simulink model "AUAV_V3_TestSensors"  (R2015a)
settings: Solver=FixedStepDiscrete  StartTime=0.0  StopTime=10.0  FixedStep=T  RelTol=1e-3
PreLoadFcn:
  | %T = 0.0025;
  | MavlinkBus;
  | mcuInit;
  | % Baro Altitude Computation
  | % =========================
  | basePressure = 98192.64;
  | baseTemp = 288.215;
  | lapseRate = -0.00198122;
  | baseHeight = 0;
undefined symbols (not defined in the file): A0, A14, A15, A2, A3, A4, A5, A6, accBiasRateLimit, apSampleTime, B0, bankCommandLimit, barAdjust, baroCutoff, baroCutTemp, baroOffset, baroScale, barTGain1, barTGain2, barTMean1, barTMean2, bda, bde, bdr, bdt, bICda, bICde, bICdr, bICdt, cubeAccelGain16405, cubeGyroGain16405, cubeMagGain16405, D0, D11, D7, D8, daLimit, data, daTrimMax, daTrimMin, deLimit, derivativesConstant, deTrimMax, deTrimMin, drLimit, drTrimMax, drTrimMin, dtLimit, dtTrimMax, dtTrimMin, F2, F3, G0, G13, G15, gaind, GS_location, gyroBiasRateLimit, IC1max, imuOffset_xacc ... (+77)
libraries: MCHP_Blockset x158, simulink x84, SLUGS_Library x31, aerolibconvert2 x6, aerolibutil x4, aerolibtransform2 x3, dspmtrx3 x2, aerolibobsolete x2
(part 11 of 23)

== system AUAV_V3_TestSensors/Trim Vals [updated 4.28.16]/Mean Filter the Transition ==
  Failsafe : Inport
  Buffer Failsafe Channel : MATLAB Function  TreatAsAtomicUnit=on
  Choose the Median [navSupport.c] [updated 5.1.16] : MCHP_Blockset/User Functions/C Function Call  ParseFilesChkbx=off  ListFunctions1=Custom Function  Function1=extern uint16_T meanFilter5(uint16_T *u1);  AddHeaderDeclaration=on  Function1Type=when block is updated (default)  Fct1BlockIn=u1  FctReturnBlockOut=on  DataCollected=0  ORDERING=None  SampleTime=-1  MCHP_MASTERLINK=|  PinDigitalInput=[]  PinDigitalOutput=[]  PinAnalogInput=[]
      | AUAV_V3_TestSensors/Microchip Master
      | AUAV V3 Board
      | Busy Flag on D2 (RA6)
  filtered : Outport
  wires:
  Choose the Median [navSupport.c] [updated 5.1.16]/1 -> filtered/1
  Failsafe/1 -> Buffer Failsafe Channel/1(latest)
  Buffer Failsafe Channel/1(history) -> Choose the Median [navSupport.c] [updated 5.1.16]/1

== system AUAV_V3_TestSensors/Update PWM Commands and Send Telemetry [updated 4.27.16]/Convert to Microseconds ==
  PWM : Inport
  Convert to Microseconds : Gain  Gain=0.2
  Data Type Conversion : DataTypeConversion  OutDataTypeStr=uint16
  uS : Outport
  wires:
  Data Type Conversion/1 -> uS/1
  PWM/1 -> Convert to Microseconds/1
  Convert to Microseconds/1 -> Data Type Conversion/1

== system AUAV_V3_TestSensors/Update PWM Commands and Send Telemetry [updated 4.27.16]/Generate PWM Signals Based on the Control Type ==
  note: Navigation Modes:
      | 2 -> PT
      | 3 -> Waypoint
      | 4 -> Mid Level
      | 8-> Sel PT
      | 9-> ISR
      | 10 -> Line Patrol
  PWM(rad) : Inport
  Pilot Console (IC) : Inport  Port=2
  isManual? : Inport  Port=3
  Nav Mode : Inport  Port=4
  Data Type Conversion : DataTypeConversion  OutDataTypeStr=uint16
  Data Type Conversion1 : DataTypeConversion  OutDataTypeStr=uint8
  If : If  NumInputs=2  IfExpression=u2 == 1  ElseIfExpressions=((u1 == 3) | (u1 == 4) | (u1 == 9) | (u1 == 10)), u1 == 2, u1 == 8  ShowElse=off  SampleTime=.01
  If  Control Type Is Manual : Subsystem  TreatAsAtomicUnit=on
  If  Control Type Is Passthrough : Subsystem  TreatAsAtomicUnit=on
  If  Control Type Is Selective Passthrough : Subsystem  TreatAsAtomicUnit=on
  "If  Control Type Is Wp, ISR, LP or  Mid Lvl Cmds" : Subsystem  TreatAsAtomicUnit=on
  Merge : Merge  Inputs=4
  PWM : Outport
  wires:
  If/1 -> If  Control Type Is Manual/Action
  If/2 -> "If  Control Type Is Wp, ISR, LP or  Mid Lvl Cmds"/Action
  If/3 -> If  Control Type Is Passthrough/Action
  If/4 -> If  Control Type Is Selective Passthrough/Action
  If  Control Type Is Manual/1(PWM) -> Merge/1
  "If  Control Type Is Wp, ISR, LP or  Mid Lvl Cmds"/1(PWM (abs)) -> Merge/2
  If  Control Type Is Passthrough/1(PWM (abs)) -> Merge/3
  If  Control Type Is Selective Passthrough/1(PWM) -> Merge/4
  PWM(rad)/1 -> "If  Control Type Is Wp, ISR, LP or  Mid Lvl Cmds"/1(PWM(rad)), If  Control Type Is Selective Passthrough/1(PWM(rad))
  Pilot Console (IC)/1 -> If  Control Type Is Manual/1(Pilot (IC)), If  Control Type Is Passthrough/1(Pilot (IC)), If  Control Type Is Selective Passthrough/2(Pilot (IC))
  Data Type Conversion/1 -> PWM/1
  isManual?/1 -> If/2
  Nav Mode/1 -> Data Type Conversion1/1
  Data Type Conversion1/1 -> If/1
  Merge/1 -> Data Type Conversion/1

== system AUAV_V3_TestSensors/Update PWM Commands and Send Telemetry [updated 4.27.16]/Send_Cmd_6DOF_HIL ==
  Enable : EnablePort
  COMP_ID : Constant  OutDataTypeStr=uint8
  Get Raw Commands : DataStoreRead  DialogController=Simulink.DDGSource  DataStoreName=mlPwmCommands  DataStoreElements=mlPwmCommands
  Get time5 : DataStoreRead  DataStoreName=time_since_boot_usec  DataStoreElements=time_since_boot_usec
  PackRawServo : MCHP_Blockset/User Functions/C Function Call  ParseFilesChkbx=on  ListFunctions1=Custom Function  Function1=uint16_t HIL_PackRawServo(uint8_t system_id, uint8_t component_id, mavlink_servo_output_raw_t mlPwmCommands ,uint32_t time_usec)  AddHeaderDeclaration=on  Function1Type=when block is updated (default)  Fct1BlockIn="system_id  , component_id  , mlPwmCommands  , time_usec"  FctReturnBlockOut=on  DataCollected="s.chksm=reshape({ '638503-Feb-2015 20:58:10','251913-Sep-2016 12:15:14','1628414-Sep-2016 10:06:29','3754120-Sep-2016 10:12:03','360317-Jun-2016 15:34:16','7114620-Sep-2016 10:38:54','954931-Aug-2016 15:03:40','295520-Sep-2016 10:30:42','268124-Jun-2016 00:23:34','556017-Jun-2016 15:34:16','963217-Jun-2016 15:34:16','1086024-Jun-2016 00:23:34','372414-Sep-2016 14:01:55','998814-Sep-2016 11:55:45','509015-Sep-2016 09:12:19'},1,15);s.File1=reshape({ '  void  newCircBuffer(CBRef cB)','  void  freeCircBuffer(CBRef* cB)','  void  freeCircBuffer(CBRef* cB)',' unsigned int  getLength(CBRef cB)','  int  readHead(CBRef cB)','  int  readTail(CBRef cB)',' unsigned char  peak(CBRef cB)',' unsigned char  readFront(CBRef cB)',' unsigned char  writeBack(CBRef cB, unsigned char data)','  void  makeEmpty(CBRef cB)','  void  printCircBuf(CBRef cB)'},1,11);s.File2=reshape({ '  void  uartBufferInit(void)','  void  __attribute__((__interrupt__, no_auto_psv)) _U4RXInterrupt(void)','  void  getGPSRawData(unsigned char* gpsBuffer)',' unsigned char  isGPSNovatel(void)'},1,4);s.File3=reshape({ '  char  hex2char(char halfhex)','  float  degMinToDeg(unsigned char degrees, float minutes)',' unsigned char  gpsUbloxSeparate(unsigned char* outStream)','  void  gpsUbloxParse(void)','  void  getGpsUbloxMainData(float* data)','  char  gpSmbl(char symbl)',' unsigned char  myTokenizer(char* stringToTokenize, char token, char * returnToken)','  void  parseRMC(unsigned char* stream)','  void  parseGGA(unsigned char* stream)',' unsigned char  getChecksum(unsigned char* sentence, unsigned char size)','  void  gpsDebugMsg(unsigned char buf)'},1,11);s.File4=reshape({ '  void  uartMavlinkBufferInit(void)','  void __attribute__((__interrupt__,__auto_psv__)) _U1RXInterrupt(void)','  uint8_t  isFinite(float s)','  void  InitParameterInterface(void)','  void  protDecodeMavlink(void)','  uint16_t  MissionInterfaceResponse(uint8_t system_id, uint8_t component_id)','  uint16_t  ParameterInterfaceResponse(uint8_t system_id, uint8_t component_id)','  uint16_t  PackHeartBeat(uint8_t system_id, uint8_t component_id)','  uint16_t  PackTextMsg(uint8_t system_id, uint8_t component_id, unsigned char buf)','  uint16_t  PackRawIMU(uint8_t system_id, uint8_t component_id, mavlink_raw_imu_t mlRawIMUData ,uint32_t time_usec)','  uint16_t  PackGpsRawInt(uint8_t system_id, uint8_t component_id, mavlink_gps_raw_int_t mlRawGpsDataInt ,uint32_t time_usec)','  uint16_t  PackScaledPressure(uint8_t system_id, uint8_t component_id, mavlink_scaled_pressure_t mlAirData ,uint32_t time_usec)','  uint16_t  PackSysStatus(uint8_t system_id, uint8_t component_id, mavlink_sys_status_t mlSysStatus)','  uint16_t  PackRawServo(uint8_t system_id, uint8_t component_id, mavlink_servo_output_raw_t mlPwmCommands ,uint32_t time_usec)','  uint16_t  HIL_PackRawServo(uint8_t system_id, uint8_t component_id, mavlink_servo_output_raw_t mlPwmCommands ,uint32_t time_usec)','  uint16_t  PackRawRC(uint8_t system_id, uint8_t component_id, mavlink_rc_channels_raw_t mlRC_Commands ,uint32_t time_usec)','  uint16_t  PackVFR_HUD(uint8_t system_id, uint8_t component_id, mavlink_vfr_hud_t mlVfr_hud ,uint32_t time_usec)','  char  sendQGCDebugMessage(const char * dbgMessage, char severity, unsigned char* bytesToAdd, char positionStart)','  void  TxN_Data_OverU1(uint16_t N)','  void  TxN_Data_OverU4(uint16_t N)'},1,20);s.File5=reshape({ '  float  myAtan2(float num, float denom)','  float  myPow(float x, float toTheN)','  float  mySqrt(float x)','  float  myAbs(float x)','  float  myAtan(float x)','  float  myAsin(float x)','  float  mySin(float x)','  float  myCos(float x)','  float  myTan(float x)','  float  myAcos(float x)','  float  myExp(float x)','  void  hugeDelay(void)','  void  smallDelay(void)','  void  tinyDelay(void)','  void  printToUart2(const char *fmt, ...)'},1,15);s.File6=reshape({ '  void  sendTelemetryMavlink(unsigned char* dataOut)','  void  uart2Init(void)','  void  gsRead(unsigned char* gsChunk)','  void  prepareTelemetryMavlink(unsigned char* dataOut)','  void  prepareTelemetryMavlink(unsigned char* dataOut)','  void  sendTelemetryMavlink(unsigned char* dataOut)','  void  copyBufferToDMA1(unsigned char size)','  void  send2GS(unsigned char* protData)','  uint8_t  clearWaypointsFrom(uint8_t startingWp)','  void  addMessageToSpiOut(mavlink_message_t* msg)'},1,10);s.File7={ '  void  populateParameterInterface(void)'};s.File8={ '  void  mavlinkInit(void)'};s.File9=reshape({ '  void  updatePWM(unsigned short * PWMData)','  void  updatePWMTrim(unsigned short PWMData, unsigned char channel)','  void  updateLoad(uint8_t mcuLoad)','  void  updateEuler(float* newEuler)','  void  updatePQR(float* newPQR)',' unsigned char  getHilOnOff(void)','  uint8_t  getLightsOnOff(void)','  uint8_t  getLightsDayNight(void)','  void  updateVISensor(uint16_t* data)','  void  updatePTZ(int16_t* ptz)'},1,10);s.File10=reshape({ '  void  updateRawADCData(int16_t* adcData)','  void  updateAirData(float* airData)','  void  updateLoadData(uint8_t load, uint16_t mvPower)','  void  updateAttitude(float * attitudeData)','  void  getGSLocation(float* altLatLon)','  void  updateTimeStamp(uint32_t timeSt)','  void  updatePosition(float * posData)','  void  updatePilotConsole(uint16_t * pilData)','  void  updateDiagnosticFl(float* diagFl)','  void  updateDiagnosticSh(int16_t* diagSh)','  void  updateBias(float * biasData)','  void  updateSensorData(float* sens)','  uint8_t  isFixValid(void)','  void  updateSensorDiag(float* diag)'},1,14);s.File11=reshape({ '  void  gpsInit(void)','  void  gpsParse(uint8_t* dataStream)','  void  updateStatus(uint8_t* completeMessage)','  void  updatePositionData(uint8_t* completeMessage)','  void  updateVelocityData(uint8_t* completeMessage)','  void  updateTimeData(uint8_t* completeMessage)','  void  getGpsMainData(float* data)','  uint32_t  CRC32Value(int32_t i)','  uint32_t  CalculateBlockCRC32(uint32_t ulCount, uint8_t *ucBuffer)','  uint16_t  charsToUint16(uint8_t* data)','  uint32_t  charsToUint32(uint8_t* data)','  float  charsToFloat(uint8_t* data)','  double  charsToDouble(uint8_t* data)'},1,13);s.File12=reshape({ '  void  getMidLevelCommands(float* commands)',' unsigned char  isApManual(uint16_t failsafe)','  float  getParamIdx(unsigned char idx)','  void  getRangeOfParams(uint8_t startIdx, uint8_t endIdx, float* parameters)','  float  getDynamic(void)','  void  getAttitude(float* attitude)','  void  getXYZ(float* xyz)','  void  getVned(float* xyz)','  uint8_t  getMaxWp(void)',' unsigned char  isWpFly(void)',' unsigned char  isPassthrough(void)','  void  setDiagnosticFloat(float * flValues)','  void  setDiagnosticShort(int16_t* shValues)','  void  getWP(unsigned char idx, float* WPpos)','  void  setLogFloat1(float * flValues)','  void  setLogFloat2(float * flValues)',' unsigned char  getApControlType(void)',' unsigned char  getPassValues(uint8_t* pasVals)','  void  setCurrentCommands(float airSpeed)','  void  getCurrentGPSPos(float* latLonAlt)','  void  setNavLong(float* values)','  void  setNavLat(float* values)','  void  setNavNav(float* values)','  void  getAccels(float * accels)','  void  getAccBias(float * bias)','  void  getRTB(uint8_t* rtb)','  void  getMobileLocation(float* loc)','  uint8_t  getNavMode(void)','  void  getISRLocation(float* loc)','  uint8_t  getISRCameraOption1(void)',' unsigned short  meanFilter5(unsigned short * values)','  uint8_t  justEnabled(uint8_t enableValue, uint8_t index)',' unsigned char  quickSort(unsigned short *arr, char elements)'},1,33);s.File13=reshape({ '  void  hilRead(unsigned char* hilChunk)','  void  hil_getRawRead(short * rawData)','  void  hil_getVned(float* vned)','  void  hil_getEuler(float* euler)','  void  hil_getRates(float* pqr)','  void  hil_getXYZ(float* xyz)',' unsigned int  hil_getTs(void)','  void  protDecodeHil(uint8_t* dataIn)'},1,8);s.File14=reshape({ '  void  cubeInit(void)','  void  getCubeData(short * cubeData)','  void  updateCubeData(void)','  int16_t  averageData(int16_t* theData, uint8_t count)',' unsigned short  write2Cube(unsigned short data2Send)','  short  convert14BitToShort(short wordData)','  short  convert12BitToShort(short wordData)',' unsigned char  isCube16405(void)'},1,8);s.File15=reshape({ '  void  uartMavlinkBufferInit(void)','  uint16_t  PackHeartBeat(uint8_t system_id, uint8_t component_id)','  uint16_t  PackRawServo(uint8_t system_id, uint8_t component_id, mavlink_servo_output_raw_t mlPwmCommands ,uint32_t time_usec)','  uint16_t  HIL_PackRawServo(uint8_t system_id, uint8_t component_id, mavlink_servo_output_raw_t mlPwmCommands ,uint32_t time_usec)','  uint16_t  PackRawRC(uint8_t system_id, uint8_t component_id, mavlink_rc_channels_raw_t mlRC_Commands, uint32_t time_usec)','  uint16_t  PackVFR_HUD(uint8_t system_id, uint8_t component_id, mavlink_vfr_hud_t mlVfr_hud, uint32_t time_usec)','  uint16_t  PackRawIMU(uint8_t system_id, uint8_t component_id, mavlink_raw_imu_t mlRawIMUData ,uint32_t time_usec)','  char  sendQGCDebugMessage(const char * dbgMessage, char severity, unsigned char* bytesToAdd, char positionStart)','  uint16_t  PackGpsRawInt(uint8_t system_id, uint8_t component_id, mavlink_gps_raw_int_t mlRawGpsDataInt, uint32_t time_usec)','  uint16_t  PackScaledPressure(uint8_t system_id, uint8_t component_id, mavlink_scaled_pressure_t mlAirData, uint32_t time_usec)','  uint16_t  PackSysStatus(uint8_t system_id, uint8_t component_id, mavlink_sys_status_t mlSysStatus)'},1,11);"  ORDERING=None  SampleTime=-1  MCHP_MASTERLINK=|  PinDigitalInput=[]  PinDigitalOutput=[]  PinAnalogInput=[]
      | AUAV_V3_TestSensors/Microchip Master
      | AUAV V3 Board
      | Busy Flag on D2 (RA6)
  SYS_ID : Constant  Value=101  OutDataTypeStr=uint8
  TX_N_Data9 : MCHP_Blockset/User Functions/C Function Call  ParseFilesChkbx=on  ListFunctions1=Custom Function  Function1=void TxN_Data_OverU4(uint16_t N)  AddHeaderDeclaration=on  Function1Type=when block is updated (default)  Fct1BlockIn=N  FctReturnBlockOut=on  DataCollected="s.chksm=reshape({ '638503-Feb-2015 20:58:10','251913-Sep-2016 12:15:14','1628414-Sep-2016 10:06:29','3754120-Sep-2016 10:12:03','360317-Jun-2016 15:34:16','7114620-Sep-2016 10:38:54','954931-Aug-2016 15:03:40','295520-Sep-2016 10:30:42','268124-Jun-2016 00:23:34','556017-Jun-2016 15:34:16','963217-Jun-2016 15:34:16','1086024-Jun-2016 00:23:34','372414-Sep-2016 14:01:55','998814-Sep-2016 11:55:45','509015-Sep-2016 09:12:19'},1,15);s.File1=reshape({ '  void  newCircBuffer(CBRef cB)','  void  freeCircBuffer(CBRef* cB)','  void  freeCircBuffer(CBRef* cB)',' unsigned int  getLength(CBRef cB)','  int  readHead(CBRef cB)','  int  readTail(CBRef cB)',' unsigned char  peak(CBRef cB)',' unsigned char  readFront(CBRef cB)',' unsigned char  writeBack(CBRef cB, unsigned char data)','  void  makeEmpty(CBRef cB)','  void  printCircBuf(CBRef cB)'},1,11);s.File2=reshape({ '  void  uartBufferInit(void)','  void  __attribute__((__interrupt__, no_auto_psv)) _U4RXInterrupt(void)','  void  getGPSRawData(unsigned char* gpsBuffer)',' unsigned char  isGPSNovatel(void)'},1,4);s.File3=reshape({ '  char  hex2char(char halfhex)','  float  degMinToDeg(unsigned char degrees, float minutes)',' unsigned char  gpsUbloxSeparate(unsigned char* outStream)','  void  gpsUbloxParse(void)','  void  getGpsUbloxMainData(float* data)','  char  gpSmbl(char symbl)',' unsigned char  myTokenizer(char* stringToTokenize, char token, char * returnToken)','  void  parseRMC(unsigned char* stream)','  void  parseGGA(unsigned char* stream)',' unsigned char  getChecksum(unsigned char* sentence, unsigned char size)','  void  gpsDebugMsg(unsigned char buf)'},1,11);s.File4=reshape({ '  void  uartMavlinkBufferInit(void)','  void __attribute__((__interrupt__,__auto_psv__)) _U1RXInterrupt(void)','  uint8_t  isFinite(float s)','  void  InitParameterInterface(void)','  void  protDecodeMavlink(void)','  uint16_t  MissionInterfaceResponse(uint8_t system_id, uint8_t component_id)','  uint16_t  ParameterInterfaceResponse(uint8_t system_id, uint8_t component_id)','  uint16_t  PackHeartBeat(uint8_t system_id, uint8_t component_id)','  uint16_t  PackTextMsg(uint8_t system_id, uint8_t component_id, unsigned char buf)','  uint16_t  PackRawIMU(uint8_t system_id, uint8_t component_id, mavlink_raw_imu_t mlRawIMUData ,uint32_t time_usec)','  uint16_t  PackGpsRawInt(uint8_t system_id, uint8_t component_id, mavlink_gps_raw_int_t mlRawGpsDataInt ,uint32_t time_usec)','  uint16_t  PackScaledPressure(uint8_t system_id, uint8_t component_id, mavlink_scaled_pressure_t mlAirData ,uint32_t time_usec)','  uint16_t  PackSysStatus(uint8_t system_id, uint8_t component_id, mavlink_sys_status_t mlSysStatus)','  uint16_t  PackRawServo(uint8_t system_id, uint8_t component_id, mavlink_servo_output_raw_t mlPwmCommands ,uint32_t time_usec)','  uint16_t  HIL_PackRawServo(uint8_t system_id, uint8_t component_id, mavlink_servo_output_raw_t mlPwmCommands ,uint32_t time_usec)','  uint16_t  PackRawRC(uint8_t system_id, uint8_t component_id, mavlink_rc_channels_raw_t mlRC_Commands ,uint32_t time_usec)','  uint16_t  PackVFR_HUD(uint8_t system_id, uint8_t component_id, mavlink_vfr_hud_t mlVfr_hud ,uint32_t time_usec)','  char  sendQGCDebugMessage(const char * dbgMessage, char severity, unsigned char* bytesToAdd, char positionStart)','  void  TxN_Data_OverU1(uint16_t N)','  void  TxN_Data_OverU4(uint16_t N)'},1,20);s.File5=reshape({ '  float  myAtan2(float num, float denom)','  float  myPow(float x, float toTheN)','  float  mySqrt(float x)','  float  myAbs(float x)','  float  myAtan(float x)','  float  myAsin(float x)','  float  mySin(float x)','  float  myCos(float x)','  float  myTan(float x)','  float  myAcos(float x)','  float  myExp(float x)','  void  hugeDelay(void)','  void  smallDelay(void)','  void  tinyDelay(void)','  void  printToUart2(const char *fmt, ...)'},1,15);s.File6=reshape({ '  void  sendTelemetryMavlink(unsigned char* dataOut)','  void  uart2Init(void)','  void  gsRead(unsigned char* gsChunk)','  void  prepareTelemetryMavlink(unsigned char* dataOut)','  void  prepareTelemetryMavlink(unsigned char* dataOut)','  void  sendTelemetryMavlink(unsigned char* dataOut)','  void  copyBufferToDMA1(unsigned char size)','  void  send2GS(unsigned char* protData)','  uint8_t  clearWaypointsFrom(uint8_t startingWp)','  void  addMessageToSpiOut(mavlink_message_t* msg)'},1,10);s.File7={ '  void  populateParameterInterface(void)'};s.File8={ '  void  mavlinkInit(void)'};s.File9=reshape({ '  void  updatePWM(unsigned short * PWMData)','  void  updatePWMTrim(unsigned short PWMData, unsigned char channel)','  void  updateLoad(uint8_t mcuLoad)','  void  updateEuler(float* newEuler)','  void  updatePQR(float* newPQR)',' unsigned char  getHilOnOff(void)','  uint8_t  getLightsOnOff(void)','  uint8_t  getLightsDayNight(void)','  void  updateVISensor(uint16_t* data)','  void  updatePTZ(int16_t* ptz)'},1,10);s.File10=reshape({ '  void  updateRawADCData(int16_t* adcData)','  void  updateAirData(float* airData)','  void  updateLoadData(uint8_t load, uint16_t mvPower)','  void  updateAttitude(float * attitudeData)','  void  getGSLocation(float* altLatLon)','  void  updateTimeStamp(uint32_t timeSt)','  void  updatePosition(float * posData)','  void  updatePilotConsole(uint16_t * pilData)','  void  updateDiagnosticFl(float* diagFl)','  void  updateDiagnosticSh(int16_t* diagSh)','  void  updateBias(float * biasData)','  void  updateSensorData(float* sens)','  uint8_t  isFixValid(void)','  void  updateSensorDiag(float* diag)'},1,14);s.File11=reshape({ '  void  gpsInit(void)','  void  gpsParse(uint8_t* dataStream)','  void  updateStatus(uint8_t* completeMessage)','  void  updatePositionData(uint8_t* completeMessage)','  void  updateVelocityData(uint8_t* completeMessage)','  void  updateTimeData(uint8_t* completeMessage)','  void  getGpsMainData(float* data)','  uint32_t  CRC32Value(int32_t i)','  uint32_t  CalculateBlockCRC32(uint32_t ulCount, uint8_t *ucBuffer)','  uint16_t  charsToUint16(uint8_t* data)','  uint32_t  charsToUint32(uint8_t* data)','  float  charsToFloat(uint8_t* data)','  double  charsToDouble(uint8_t* data)'},1,13);s.File12=reshape({ '  void  getMidLevelCommands(float* commands)',' unsigned char  isApManual(uint16_t failsafe)','  float  getParamIdx(unsigned char idx)','  void  getRangeOfParams(uint8_t startIdx, uint8_t endIdx, float* parameters)','  float  getDynamic(void)','  void  getAttitude(float* attitude)','  void  getXYZ(float* xyz)','  void  getVned(float* xyz)','  uint8_t  getMaxWp(void)',' unsigned char  isWpFly(void)',' unsigned char  isPassthrough(void)','  void  setDiagnosticFloat(float * flValues)','  void  setDiagnosticShort(int16_t* shValues)','  void  getWP(unsigned char idx, float* WPpos)','  void  setLogFloat1(float * flValues)','  void  setLogFloat2(float * flValues)',' unsigned char  getApControlType(void)',' unsigned char  getPassValues(uint8_t* pasVals)','  void  setCurrentCommands(float airSpeed)','  void  getCurrentGPSPos(float* latLonAlt)','  void  setNavLong(float* values)','  void  setNavLat(float* values)','  void  setNavNav(float* values)','  void  getAccels(float * accels)','  void  getAccBias(float * bias)','  void  getRTB(uint8_t* rtb)','  void  getMobileLocation(float* loc)','  uint8_t  getNavMode(void)','  void  getISRLocation(float* loc)','  uint8_t  getISRCameraOption1(void)',' unsigned short  meanFilter5(unsigned short * values)','  uint8_t  justEnabled(uint8_t enableValue, uint8_t index)',' unsigned char  quickSort(unsigned short *arr, char elements)'},1,33);s.File13=reshape({ '  void  hilRead(unsigned char* hilChunk)','  void  hil_getRawRead(short * rawData)','  void  hil_getVned(float* vned)','  void  hil_getEuler(float* euler)','  void  hil_getRates(float* pqr)','  void  hil_getXYZ(float* xyz)',' unsigned int  hil_getTs(void)','  void  protDecodeHil(uint8_t* dataIn)'},1,8);s.File14=reshape({ '  void  cubeInit(void)','  void  getCubeData(short * cubeData)','  void  updateCubeData(void)','  int16_t  averageData(int16_t* theData, uint8_t count)',' unsigned short  write2Cube(unsigned short data2Send)','  short  convert14BitToShort(short wordData)','  short  convert12BitToShort(short wordData)',' unsigned char  isCube16405(void)'},1,8);s.File15=reshape({ '  void  uartMavlinkBufferInit(void)','  uint16_t  PackHeartBeat(uint8_t system_id, uint8_t component_id)','  uint16_t  PackRawServo(uint8_t system_id, uint8_t component_id, mavlink_servo_output_raw_t mlPwmCommands ,uint32_t time_usec)','  uint16_t  HIL_PackRawServo(uint8_t system_id, uint8_t component_id, mavlink_servo_output_raw_t mlPwmCommands ,uint32_t time_usec)','  uint16_t  PackRawRC(uint8_t system_id, uint8_t component_id, mavlink_rc_channels_raw_t mlRC_Commands, uint32_t time_usec)','  uint16_t  PackVFR_HUD(uint8_t system_id, uint8_t component_id, mavlink_vfr_hud_t mlVfr_hud, uint32_t time_usec)','  uint16_t  PackRawIMU(uint8_t system_id, uint8_t component_id, mavlink_raw_imu_t mlRawIMUData ,uint32_t time_usec)','  char  sendQGCDebugMessage(const char * dbgMessage, char severity, unsigned char* bytesToAdd, char positionStart)','  uint16_t  PackGpsRawInt(uint8_t system_id, uint8_t component_id, mavlink_gps_raw_int_t mlRawGpsDataInt, uint32_t time_usec)','  uint16_t  PackScaledPressure(uint8_t system_id, uint8_t component_id, mavlink_scaled_pressure_t mlAirData, uint32_t time_usec)','  uint16_t  PackSysStatus(uint8_t system_id, uint8_t component_id, mavlink_sys_status_t mlSysStatus)'},1,11);"  ORDERING=None  SampleTime=-1  MCHP_MASTERLINK=|  PinDigitalInput=[]  PinDigitalOutput=[]  PinAnalogInput=[]
      | AUAV_V3_TestSensors/Microchip Master
      | AUAV V3 Board
      | Busy Flag on D2 (RA6)
  wires:
  PackRawServo/1 -> TX_N_Data9/1
  SYS_ID/1 -> PackRawServo/1
  Get time5/1 -> ?
  Get Raw Commands/1 -> PackRawServo/3
  COMP_ID/1 -> PackRawServo/2

== system AUAV_V3_TestSensors/Update PWM Commands and Send Telemetry [updated 4.27.16]/Send_Cmd_X_Plane_HIL ==
  Enable : EnablePort
  PackRawServo : MCHP_Blockset/User Functions/C Function Call  ParseFilesChkbx=on  ListFunctions1=Custom Function  Function1=uint16_t send_HILSIM_outputs(void)  AddHeaderDeclaration=on  Function1Type=when block is updated (default)  FctReturnBlockOut=on  Fct1BlockOut=N  DataCollected="s.chksm=reshape({ '638527-Oct-2016 19:19:54','255931-Oct-2016 16:54:23','1693602-Nov-2016 16:03:49','4463902-Nov-2016 15:21:25','369131-Oct-2016 16:54:23','7293731-Oct-2016 16:54:23','954931-Oct-2016 16:54:23','296731-Oct-2016 16:54:23','278131-Oct-2016 16:54:23','673001-Nov-2016 10:31:31','963231-Oct-2016 16:54:23','1122631-Oct-2016 16:54:23','372402-Nov-2016 16:11:38','998831-Oct-2016 16:54:23','4195003-Nov-2016 08:56:40','549731-Oct-2016 16:54:23'},1,16);s.File1=reshape({ '  void  newCircBuffer(CBRef cB)','  void  freeCircBuffer(CBRef* cB)','  void  freeCircBuffer(CBRef* cB)',' unsigned int  getLength(CBRef cB)','  int  readHead(CBRef cB)','  int  readTail(CBRef cB)',' unsigned char  peak(CBRef cB)',' unsigned char  readFront(CBRef cB)',' unsigned char  writeBack(CBRef cB, unsigned char data)','  void  makeEmpty(CBRef cB)','  void  printCircBuf(CBRef cB)'},1,11);s.File2=reshape({ '  void  uartBufferInit(void)','  void  __attribute__((__interrupt__, no_auto_psv)) _U4RXInterrupt(void)','  void  getGPSRawData(unsigned char* gpsBuffer)',' unsigned char  isGPSNovatel(void)'},1,4);s.File3=reshape({ 'extern  void  TxN_Data_OverU1(uint16_t N)','extern  uint16_t  PackTextMsg(uint8_t system_id, uint8_t component_id, unsigned char buf)','  char  hex2char(char halfhex)','  float  degMinToDeg(unsigned char degrees, float minutes)',' unsigned char  gpsUbloxSeparate(unsigned char* outStream)','  void  gpsUbloxParse(void)','  void  getGpsUbloxMainData(float* data)','  void  getGpsUbloxData(float* data)','  char  gpSmbl(char symbl)',' unsigned char  myTokenizer(char* stringToTokenize, char token, char * returnToken)','  void  parseRMC(unsigned char* stream)','  void  parseGGA(unsigned char* stream)',' unsigned char  getChecksum(unsigned char* sentence, unsigned char size)','  void  gpsDebugMsg(unsigned char buf)'},1,14);s.File4=reshape({ '  void  uartMavlinkBufferInit(void)','  void __attribute__((__interrupt__,__auto_psv__)) _U1RXInterrupt(void)','  uint8_t  isFinite(float s)','  void  InitParameterInterface(void)','  void  protDecodeMavlink(void)','  uint16_t  MissionInterfaceResponse(uint8_t system_id, uint8_t component_id)','  uint16_t  ParameterInterfaceResponse(uint8_t system_id, uint8_t component_id)','  uint16_t  PackHeartBeat(uint8_t system_id, uint8_t component_id)','  uint16_t  PackTextMsg(uint8_t system_id, uint8_t component_id, unsigned char buf)','  uint16_t  PackRawIMU(uint8_t system_id, uint8_t component_id, mavlink_raw_imu_t mlRawIMUData ,uint32_t time_usec)','  uint16_t  PackRawAttitude(uint8_t system_id, uint8_t component_id, mavlink_attitude_t mlAttitudeData ,uint32_t time_usec)','  uint16_t  PackRawNavigation(uint8_t system_id, uint8_t component_id, mavlink_slugs_navigation_t mlNavigation, uint32_t time_usec)','  uint16_t  PackPosXYZ_Sol(uint8_t system_id, uint8_t component_id, mavlink_local_position_ned_t mlLocalPositionSol ,uint32_t time_usec)','  uint16_t  PackGpsRawInt(uint8_t system_id, uint8_t component_id, mavlink_gps_raw_int_t mlRawGpsDataInt ,uint32_t time_usec)','  uint16_t  PackScaledPressure(uint8_t system_id, uint8_t component_id, mavlink_scaled_pressure_t mlAirData ,uint32_t time_usec)','  uint16_t  PackSysStatus(uint8_t system_id, uint8_t component_id, mavlink_sys_status_t mlSysStatus)','  uint16_t  PackRawServo(uint8_t system_id, uint8_t component_id, mavlink_servo_output_raw_t mlPwmCommands ,uint32_t time_usec)','  uint16_t  HIL_PackRawServo(uint8_t system_id, uint8_t component_id, mavlink_servo_output_raw_t mlPwmCommands ,uint32_t time_usec)','  uint16_t  PackRawRC(uint8_t system_id, uint8_t component_id, mavlink_rc_channels_raw_t mlRC_Commands ,uint32_t time_usec)','  uint16_t  PackVFR_HUD(uint8_t system_id, uint8_t component_id, mavlink_vfr_hud_t mlVfr_hud ,uint32_t time_usec)','  char  sendQGCDebugMessage(const char * dbgMessage, char severity, unsigned char* bytesToAdd, char positionStart)','  void  TxN_Data_OverU1(uint16_t N)','  void  TxN_Data_OverU4(uint16_t N)'},1,23);s.File5=reshape({ '  float  myAtan2(float num, float denom)','  float  myPow(float x, float toTheN)','  float  mySqrt(float x)','  float  myAbs(float x)','  float  myAtan(float x)','  float  myAsin(float x)','  float  mySin(float x)','  float  myCos(float x)','  float  myTan(float x)','  float  myAcos(float x)','  float  myExp(float x)','  void  hugeDelay(void)','  void  smallDelay(void)','  void  tinyDelay(void)'},1,14);s.File6=reshape({ '  void  sendTelemetryMavlink(unsigned char* dataOut)','  void  uart2Init(void)','  void  gsRead(unsigned char* gsChunk)','  void  prepareTelemetryMavlink(unsigned char* dataOut)','  void  prepareTelemetryMavlink(unsigned char* dataOut)','  void  sendTelemetryMavlink(unsigned char* dataOut)','  void  copyBufferToDMA1(unsigned char size)','  void  send2GS(unsigned char* protData)','  uint8_t  clearWaypointsFrom(uint8_t startingWp)','  void  addMessageToSpiOut(mavlink_message_t* msg)'},1,10);s.File7={ '  void  populateParameterInterface(void)'};s.File8={ '  void  mavlinkInit(void)'};s.File9=reshape({ '  void  updatePWM(unsigned short * PWMData)','  void  updatePWMTrim(unsigned short PWMData, unsigned char channel)','  void  updateLoad(uint8_t mcuLoad)','  void  updateEuler(float* newEuler)','  void  updatePQR(float* newPQR)',' unsigned char  getHilOnOff(void)','  uint8_t  getLightsOnOff(void)','  uint8_t  getLightsDayNight(void)','  void  updateVISensor(uint16_t* data)','  void  updatePTZ(int16_t* ptz)'},1,10);s.File10=reshape({ 'extern  float  myPow(float x, float toTheN)','  void  updateRawADCData(int16_t* adcData)','  void  updateAirData(float* airData)','  void  updateLoadData(uint8_t load, uint16_t mvPower)','  void  updateAttitude(float * attitudeData)','  void  getGSLocation(float* altLatLon)','  void  updateTimeStamp(uint32_t timeSt)','  void  updatePosition(float * posData)','  void  updatePilotConsole(uint16_t * pilData)','  void  updateDiagnosticFl(float* diagFl)','  void  updateDiagnosticSh(int16_t* diagSh)','  void  updateBias(float * biasData)','  void  updateSensorData(float* sens)','  uint8_t  isFixValid(void)','  void  updateSensorDiag(float* diag)'},1,15);s.File11=reshape({ '  void  gpsInit(void)','  void  gpsParse(uint8_t* dataStream)','  void  updateStatus(uint8_t* completeMessage)','  void  updatePositionData(uint8_t* completeMessage)','  void  updateVelocityData(uint8_t* completeMessage)','  void  updateTimeData(uint8_t* completeMessage)','  void  getGpsMainData(float* data)','  uint32_t  CRC32Value(int32_t i)','  uint32_t  CalculateBlockCRC32(uint32_t ulCount, uint8_t *ucBuffer)','  uint16_t  charsToUint16(uint8_t* data)','  uint32_t  charsToUint32(uint8_t* data)','  float  charsToFloat(uint8_t* data)','  double  charsToDouble(uint8_t* data)'},1,13);s.File12=reshape({ '  void  getMidLevelCommands(float* commands)',' unsigned char  isApManual(uint16_t failsafe)','  float  getParamIdx(unsigned char idx)','  void  getRangeOfParams(uint8_t startIdx, uint8_t endIdx, float* parameters)','  float  getDynamic(void)','  void  getAttitude(float* attitude)','  void  getXYZ(float* xyz)','  void  getVned(float* xyz)','  uint8_t  getMaxWp(void)',' unsigned char  isWpFly(void)',' unsigned char  isPassthrough(void)','  void  setDiagnosticFloat(float * flValues)','  void  setDiagnosticShort(int16_t* shValues)','  void  getWP(unsigned char idx, float* WPpos)','  void  setLogFloat1(float * flValues)','  void  setLogFloat2(float * flValues)',' unsigned char  getApControlType(void)',' unsigned char  getPassValues(uint8_t* pasVals)','  void  setCurrentCommands(float airSpeed)','  void  getCurrentGPSPos(float* latLonAlt)','  void  setNavLong(float* values)','  void  setNavLat(float* values)','  void  setNavNav(float* values)','  void  getAccels(float * accels)','  void  getAccBias(float * bias)','  void  getRTB(uint8_t* rtb)','  void  getMobileLocation(float* loc)','  uint8_t  getNavMode(void)','  void  getISRLocation(float* loc)','  uint8_t  getISRCameraOption1(void)',' unsigned short  meanFilter5(unsigned short * values)','  uint8_t  justEnabled(uint8_t enableValue, uint8_t index)',' unsigned char  quickSort(unsigned short *arr, char elements)'},1,33);s.File13=reshape({ '  void  hilRead(unsigned char* hilChunk)','  void  hil_getRawRead(short * rawData)','  void  hil_getVned(float* vned)','  void  hil_getEuler(float* euler)','  void  hil_getRates(float* pqr)','  void  hil_getXYZ(float* xyz)',' unsigned int  hil_getTs(void)','  void  protDecodeHil(uint8_t* dataIn)'},1,8);s.File14=reshape({ '  void  cubeInit(void)','  void  getCubeData(short * cubeData)','  void  updateCubeData(void)','  int16_t  averageData(int16_t* theData, uint8_t count)',' unsigned short  write2Cube(unsigned short data2Send)','  short  convert14BitToShort(short wordData)','  short  convert12BitToShort(short wordData)',' unsigned char  isCube16405(void)'},1,8);s.File15=reshape({ '  void  udb_background_trigger(background_callback callback)','  void  gpsoutline(const char* message)','  void  gpsoutbin(int16_t length, const uint8_t* msg)','  void  commit_bodyrate_data(void)','  void  gps_startup_sequence(int16_t gpscount)','  void  nmea_passthru(uint8_t gpschar)','  void  udb_background_trigger(background_callback callback)','  void  gps_update_basic_data(void)','  void  gps_commit_data(void)','  void  commit_bodyrate_data(void)','  void  HILSIM_saturate(uint16_t size , int16_t vector[3])','  void  HILSIM_set_gplane(void)','  void  HILSIM_set_omegagyro(void)','  void  init_gps_ubx(void)','  void  gpsoutbin(int16_t length, const uint8_t msg[])','  void  gpsoutline(const char *message)','  int16_t  udb_gps_callback_get_byte_to_send(void)','  void  udb_gps_callback_received_byte(uint8_t rxchar)','  uint16_t  send_HILSIM_outputs(void)'},1,19);s.File16=reshape({ '  void  uartMavlinkBufferInit(void)','  uint16_t  PackHeartBeat(uint8_t system_id, uint8_t component_id)','  uint16_t  PackRawServo(uint8_t system_id, uint8_t component_id, mavlink_servo_output_raw_t mlPwmCommands ,uint32_t time_usec)','  uint16_t  HIL_PackRawServo(uint8_t system_id, uint8_t component_id, mavlink_servo_output_raw_t mlPwmCommands ,uint32_t time_usec)','  uint16_t  PackRawRC(uint8_t system_id, uint8_t component_id, mavlink_rc_channels_raw_t mlRC_Commands, uint32_t time_usec)','  uint16_t  PackVFR_HUD(uint8_t system_id, uint8_t component_id, mavlink_vfr_hud_t mlVfr_hud, uint32_t time_usec)','  uint16_t  PackRawIMU(uint8_t system_id, uint8_t component_id, mavlink_raw_imu_t mlRawIMUData ,uint32_t time_usec)','  uint16_t  PackRawAttitude(uint8_t system_id, uint8_t component_id, mavlink_attitude_t mlAttitudeData ,uint32_t time_usec)','  uint16_t  PackPosXYZ_Sol(uint8_t system_id, uint8_t component_id, mavlink_local_position_ned_t mlLocalPositionSol ,uint32_t time_usec)','  uint16_t  PackRawNavigation(uint8_t system_id, uint8_t component_id, mavlink_slugs_navigation_t mlNavigation, uint32_t time_usec)','  char  sendQGCDebugMessage(const char * dbgMessage, char severity, unsigned char* bytesToAdd, char positionStart)','  uint16_t  PackGpsRawInt(uint8_t system_id, uint8_t component_id, mavlink_gps_raw_int_t mlRawGpsDataInt, uint32_t time_usec)','  uint16_t  PackScaledPressure(uint8_t system_id, uint8_t component_id, mavlink_scaled_pressure_t mlAirData, uint32_t time_usec)','  uint16_t  PackSysStatus(uint8_t system_id, uint8_t component_id, mavlink_sys_status_t mlSysStatus)'},1,14);"  ORDERING=None  SampleTime=-1  MCHP_MASTERLINK=|  PinDigitalInput=[]  PinDigitalOutput=[]  PinAnalogInput=[]
      | AUAV_V3_TestSensors/Microchip Master
      | AUAV V3 Board
      | Busy Flag on D2 (RA6)
  TX_N_Data9 : MCHP_Blockset/User Functions/C Function Call  ParseFilesChkbx=on  ListFunctions1=Custom Function  Function1=void TxN_Data_OverU4(uint16_t N)  AddHeaderDeclaration=on  Function1Type=when block is updated (default)  Fct1BlockIn=N  FctReturnBlockOut=on  DataCollected="s.chksm=reshape({ '638527-Oct-2016 19:19:54','255931-Oct-2016 16:54:23','1693602-Nov-2016 16:03:49','4463902-Nov-2016 15:21:25','369131-Oct-2016 16:54:23','7293731-Oct-2016 16:54:23','954931-Oct-2016 16:54:23','296731-Oct-2016 16:54:23','278131-Oct-2016 16:54:23','673001-Nov-2016 10:31:31','963231-Oct-2016 16:54:23','1122631-Oct-2016 16:54:23','372402-Nov-2016 16:11:38','998831-Oct-2016 16:54:23','4189902-Nov-2016 16:03:46','549731-Oct-2016 16:54:23'},1,16);s.File1=reshape({ '  void  newCircBuffer(CBRef cB)','  void  freeCircBuffer(CBRef* cB)','  void  freeCircBuffer(CBRef* cB)',' unsigned int  getLength(CBRef cB)','  int  readHead(CBRef cB)','  int  readTail(CBRef cB)',' unsigned char  peak(CBRef cB)',' unsigned char  readFront(CBRef cB)',' unsigned char  writeBack(CBRef cB, unsigned char data)','  void  makeEmpty(CBRef cB)','  void  printCircBuf(CBRef cB)'},1,11);s.File2=reshape({ '  void  uartBufferInit(void)','  void  __attribute__((__interrupt__, no_auto_psv)) _U4RXInterrupt(void)','  void  getGPSRawData(unsigned char* gpsBuffer)',' unsigned char  isGPSNovatel(void)'},1,4);s.File3=reshape({ 'extern  void  TxN_Data_OverU1(uint16_t N)','extern  uint16_t  PackTextMsg(uint8_t system_id, uint8_t component_id, unsigned char buf)','  char  hex2char(char halfhex)','  float  degMinToDeg(unsigned char degrees, float minutes)',' unsigned char  gpsUbloxSeparate(unsigned char* outStream)','  void  gpsUbloxParse(void)','  void  getGpsUbloxMainData(float* data)','  void  getGpsUbloxData(float* data)','  char  gpSmbl(char symbl)',' unsigned char  myTokenizer(char* stringToTokenize, char token, char * returnToken)','  void  parseRMC(unsigned char* stream)','  void  parseGGA(unsigned char* stream)',' unsigned char  getChecksum(unsigned char* sentence, unsigned char size)','  void  gpsDebugMsg(unsigned char buf)'},1,14);s.File4=reshape({ '  void  uartMavlinkBufferInit(void)','  void __attribute__((__interrupt__,__auto_psv__)) _U1RXInterrupt(void)','  uint8_t  isFinite(float s)','  void  InitParameterInterface(void)','  void  protDecodeMavlink(void)','  uint16_t  MissionInterfaceResponse(uint8_t system_id, uint8_t component_id)','  uint16_t  ParameterInterfaceResponse(uint8_t system_id, uint8_t component_id)','  uint16_t  PackHeartBeat(uint8_t system_id, uint8_t component_id)','  uint16_t  PackTextMsg(uint8_t system_id, uint8_t component_id, unsigned char buf)','  uint16_t  PackRawIMU(uint8_t system_id, uint8_t component_id, mavlink_raw_imu_t mlRawIMUData ,uint32_t time_usec)','  uint16_t  PackRawAttitude(uint8_t system_id, uint8_t component_id, mavlink_attitude_t mlAttitudeData ,uint32_t time_usec)','  uint16_t  PackRawNavigation(uint8_t system_id, uint8_t component_id, mavlink_slugs_navigation_t mlNavigation, uint32_t time_usec)','  uint16_t  PackPosXYZ_Sol(uint8_t system_id, uint8_t component_id, mavlink_local_position_ned_t mlLocalPositionSol ,uint32_t time_usec)','  uint16_t  PackGpsRawInt(uint8_t system_id, uint8_t component_id, mavlink_gps_raw_int_t mlRawGpsDataInt ,uint32_t time_usec)','  uint16_t  PackScaledPressure(uint8_t system_id, uint8_t component_id, mavlink_scaled_pressure_t mlAirData ,uint32_t time_usec)','  uint16_t  PackSysStatus(uint8_t system_id, uint8_t component_id, mavlink_sys_status_t mlSysStatus)','  uint16_t  PackRawServo(uint8_t system_id, uint8_t component_id, mavlink_servo_output_raw_t mlPwmCommands ,uint32_t time_usec)','  uint16_t  HIL_PackRawServo(uint8_t system_id, uint8_t component_id, mavlink_servo_output_raw_t mlPwmCommands ,uint32_t time_usec)','  uint16_t  PackRawRC(uint8_t system_id, uint8_t component_id, mavlink_rc_channels_raw_t mlRC_Commands ,uint32_t time_usec)','  uint16_t  PackVFR_HUD(uint8_t system_id, uint8_t component_id, mavlink_vfr_hud_t mlVfr_hud ,uint32_t time_usec)','  char  sendQGCDebugMessage(const char * dbgMessage, char severity, unsigned char* bytesToAdd, char positionStart)','  void  TxN_Data_OverU1(uint16_t N)','  void  TxN_Data_OverU4(uint16_t N)'},1,23);s.File5=reshape({ '  float  myAtan2(float num, float denom)','  float  myPow(float x, float toTheN)','  float  mySqrt(float x)','  float  myAbs(float x)','  float  myAtan(float x)','  float  myAsin(float x)','  float  mySin(float x)','  float  myCos(float x)','  float  myTan(float x)','  float  myAcos(float x)','  float  myExp(float x)','  void  hugeDelay(void)','  void  smallDelay(void)','  void  tinyDelay(void)'},1,14);s.File6=reshape({ '  void  sendTelemetryMavlink(unsigned char* dataOut)','  void  uart2Init(void)','  void  gsRead(unsigned char* gsChunk)','  void  prepareTelemetryMavlink(unsigned char* dataOut)','  void  prepareTelemetryMavlink(unsigned char* dataOut)','  void  sendTelemetryMavlink(unsigned char* dataOut)','  void  copyBufferToDMA1(unsigned char size)','  void  send2GS(unsigned char* protData)','  uint8_t  clearWaypointsFrom(uint8_t startingWp)','  void  addMessageToSpiOut(mavlink_message_t* msg)'},1,10);s.File7={ '  void  populateParameterInterface(void)'};s.File8={ '  void  mavlinkInit(void)'};s.File9=reshape({ '  void  updatePWM(unsigned short * PWMData)','  void  updatePWMTrim(unsigned short PWMData, unsigned char channel)','  void  updateLoad(uint8_t mcuLoad)','  void  updateEuler(float* newEuler)','  void  updatePQR(float* newPQR)',' unsigned char  getHilOnOff(void)','  uint8_t  getLightsOnOff(void)','  uint8_t  getLightsDayNight(void)','  void  updateVISensor(uint16_t* data)','  void  updatePTZ(int16_t* ptz)'},1,10);s.File10=reshape({ 'extern  float  myPow(float x, float toTheN)','  void  updateRawADCData(int16_t* adcData)','  void  updateAirData(float* airData)','  void  updateLoadData(uint8_t load, uint16_t mvPower)','  void  updateAttitude(float * attitudeData)','  void  getGSLocation(float* altLatLon)','  void  updateTimeStamp(uint32_t timeSt)','  void  updatePosition(float * posData)','  void  updatePilotConsole(uint16_t * pilData)','  void  updateDiagnosticFl(float* diagFl)','  void  updateDiagnosticSh(int16_t* diagSh)','  void  updateBias(float * biasData)','  void  updateSensorData(float* sens)','  uint8_t  isFixValid(void)','  void  updateSensorDiag(float* diag)'},1,15);s.File11=reshape({ '  void  gpsInit(void)','  void  gpsParse(uint8_t* dataStream)','  void  updateStatus(uint8_t* completeMessage)','  void  updatePositionData(uint8_t* completeMessage)','  void  updateVelocityData(uint8_t* completeMessage)','  void  updateTimeData(uint8_t* completeMessage)','  void  getGpsMainData(float* data)','  uint32_t  CRC32Value(int32_t i)','  uint32_t  CalculateBlockCRC32(uint32_t ulCount, uint8_t *ucBuffer)','  uint16_t  charsToUint16(uint8_t* data)','  uint32_t  charsToUint32(uint8_t* data)','  float  charsToFloat(uint8_t* data)','  double  charsToDouble(uint8_t* data)'},1,13);s.File12=reshape({ '  void  getMidLevelCommands(float* commands)',' unsigned char  isApManual(uint16_t failsafe)','  float  getParamIdx(unsigned char idx)','  void  getRangeOfParams(uint8_t startIdx, uint8_t endIdx, float* parameters)','  float  getDynamic(void)','  void  getAttitude(float* attitude)','  void  getXYZ(float* xyz)','  void  getVned(float* xyz)','  uint8_t  getMaxWp(void)',' unsigned char  isWpFly(void)',' unsigned char  isPassthrough(void)','  void  setDiagnosticFloat(float * flValues)','  void  setDiagnosticShort(int16_t* shValues)','  void  getWP(unsigned char idx, float* WPpos)','  void  setLogFloat1(float * flValues)','  void  setLogFloat2(float * flValues)',' unsigned char  getApControlType(void)',' unsigned char  getPassValues(uint8_t* pasVals)','  void  setCurrentCommands(float airSpeed)','  void  getCurrentGPSPos(float* latLonAlt)','  void  setNavLong(float* values)','  void  setNavLat(float* values)','  void  setNavNav(float* values)','  void  getAccels(float * accels)','  void  getAccBias(float * bias)','  void  getRTB(uint8_t* rtb)','  void  getMobileLocation(float* loc)','  uint8_t  getNavMode(void)','  void  getISRLocation(float* loc)','  uint8_t  getISRCameraOption1(void)',' unsigned short  meanFilter5(unsigned short * values)','  uint8_t  justEnabled(uint8_t enableValue, uint8_t index)',' unsigned char  quickSort(unsigned short *arr, char elements)'},1,33);s.File13=reshape({ '  void  hilRead(unsigned char* hilChunk)','  void  hil_getRawRead(short * rawData)','  void  hil_getVned(float* vned)','  void  hil_getEuler(float* euler)','  void  hil_getRates(float* pqr)','  void  hil_getXYZ(float* xyz)',' unsigned int  hil_getTs(void)','  void  protDecodeHil(uint8_t* dataIn)'},1,8);s.File14=reshape({ '  void  cubeInit(void)','  void  getCubeData(short * cubeData)','  void  updateCubeData(void)','  int16_t  averageData(int16_t* theData, uint8_t count)',' unsigned short  write2Cube(unsigned short data2Send)','  short  convert14BitToShort(short wordData)','  short  convert12BitToShort(short wordData)',' unsigned char  isCube16405(void)'},1,8);s.File15=reshape({ '  void  udb_background_trigger(background_callback callback)','  void  gpsoutline(const char* message)','  void  gpsoutbin(int16_t length, const uint8_t* msg)','  void  commit_bodyrate_data(void)','  void  gps_startup_sequence(int16_t gpscount)','  void  nmea_passthru(uint8_t gpschar)','  void  udb_background_trigger(background_callback callback)','  void  gps_update_basic_data(void)','  void  gps_commit_data(void)','  void  commit_bodyrate_data(void)','  void  HILSIM_saturate(uint16_t size , int16_t vector[3])','  void  HILSIM_set_gplane(void)','  void  HILSIM_set_omegagyro(void)','  void  init_gps_ubx(void)','  void  gpsoutbin(int16_t length, const uint8_t msg[])','  void  gpsoutline(const char *message)','  int16_t  udb_gps_callback_get_byte_to_send(void)','  void  udb_gps_callback_received_byte(uint8_t rxchar)','  int16_t  send_HILSIM_outputs(void)'},1,19);s.File16=reshape({ '  void  uartMavlinkBufferInit(void)','  uint16_t  PackHeartBeat(uint8_t system_id, uint8_t component_id)','  uint16_t  PackRawServo(uint8_t system_id, uint8_t component_id, mavlink_servo_output_raw_t mlPwmCommands ,uint32_t time_usec)','  uint16_t  HIL_PackRawServo(uint8_t system_id, uint8_t component_id, mavlink_servo_output_raw_t mlPwmCommands ,uint32_t time_usec)','  uint16_t  PackRawRC(uint8_t system_id, uint8_t component_id, mavlink_rc_channels_raw_t mlRC_Commands, uint32_t time_usec)','  uint16_t  PackVFR_HUD(uint8_t system_id, uint8_t component_id, mavlink_vfr_hud_t mlVfr_hud, uint32_t time_usec)','  uint16_t  PackRawIMU(uint8_t system_id, uint8_t component_id, mavlink_raw_imu_t mlRawIMUData ,uint32_t time_usec)','  uint16_t  PackRawAttitude(uint8_t system_id, uint8_t component_id, mavlink_attitude_t mlAttitudeData ,uint32_t time_usec)','  uint16_t  PackPosXYZ_Sol(uint8_t system_id, uint8_t component_id, mavlink_local_position_ned_t mlLocalPositionSol ,uint32_t time_usec)','  uint16_t  PackRawNavigation(uint8_t system_id, uint8_t component_id, mavlink_slugs_navigation_t mlNavigation, uint32_t time_usec)','  char  sendQGCDebugMessage(const char * dbgMessage, char severity, unsigned char* bytesToAdd, char positionStart)','  uint16_t  PackGpsRawInt(uint8_t system_id, uint8_t component_id, mavlink_gps_raw_int_t mlRawGpsDataInt, uint32_t time_usec)','  uint16_t  PackScaledPressure(uint8_t system_id, uint8_t component_id, mavlink_scaled_pressure_t mlAirData, uint32_t time_usec)','  uint16_t  PackSysStatus(uint8_t system_id, uint8_t component_id, mavlink_sys_status_t mlSysStatus)'},1,14);"  ORDERING=None  SampleTime=-1  MCHP_MASTERLINK=|  PinDigitalInput=[]  PinDigitalOutput=[]  PinAnalogInput=[]
      | AUAV_V3_TestSensors/Microchip Master
      | AUAV V3 Board
      | Busy Flag on D2 (RA6)
  wires:
  PackRawServo/1 -> TX_N_Data9/1
